simulink model "Backhoe_TiltCyl_Valve_Variants"  (R2016a)
settings: Solver=ode23t  StartTime=0.0  StopTime=60  MaxStep=0.01  RelTol=1e-3
PostLoadFcn:
  | warning off Simulink:Engine:UsingDefaultMaxStepSize
  | warning off Simulink:blocks:MatchingFromNotFound
  | warning off Simulink:Engine:SaveWithParameterizedLinks_Warning
  | warning off Simulink:Engine:SolverMinStepNonlinearIterWarnForDAE
model workspace (MAT data in the model file):
  cylinderGray = [0.6 0.6 0.6]
  darkOrange = [0.8 0.5 0]
  glassBlue = [0.2 0.2 1]
  gray = [0.3 0.3 0.3]
  orange = [0.8 0.65 0]
  pistonGray = [0.4 0.4 0.4]
  rhoGlass = 2500
  rhoRubber = 1500
  rhoSteel = 7800
  tireBlack = [0.1 0.1 0.1]
  wheelGray = [0.6 0.6 0.6]
  yellow = [0.8 0.8 0]
undefined symbols (not defined in the file or in its folder): BH_Param, sigbuilder_block, X, Y, Z
libraries: sm_lib x54, fl_lib x15, Backhoe_Lib x15, nesl_utility x7, sh_lib x4, Custom_Valve_Choices_Lib x1
(part 1 of 2)
Description:
  | Copyright 2014-2016 The MathWorks, Inc.
settings Model: Creator=smiller  LastModifiedBy=smiller
settings DataIOCC: LimitDataPoints=on  SaveFormat=Array
settings OptimizationCC: ExpressionDepthLimit=2147483647
settings DebuggingCC: UnderspecifiedInitializationDetection=Classic  MergeDetectMultiDrivingBlocksExec=none  SolverPrmCheckMsg=warning  AllowSymbolicDim=off  StateNameClashWarn=warning
settings HardwareCC: ProdBitPerPointer=32  ProdLargestAtomicFloat=None  ProdIntDivRoundTo=Undefined  ProdEndianess=Unspecified  ProdWordSize=32  ProdHWDeviceType=32-bit Generic
settings ModelReferenceCC: PropagateSignalLabelsOutOfModel=off
settings ConfigComp: CovModelRefEnable=Off  CovSFcnEnable=off
settings ConfigurationSet: Description=SimMechanics 2G
settings ExplorerConfigSet: InternalSimMechanicsExplorerSettings="<ExplorerConfiguration><canonicalview>default</canonicalview><TilePanel><TileInfo><Tiles Columns=\"1\" Count=\"1\" Rows=\"1\"><Column Left=\"2\" Weight=\"1\"/><Column Left=\"516\"/><Row Top=\"2\" Weight=\"1\"/><Row Top=\"405\"/><Tile Height=\"1\" Width=\"1\" X=\"0\" Y=\"0\"/></Tiles></TileInfo><SceneInfo><SceneViewer><BGColor><R>0.60000002384185791</R><G>0.60000002384185791</G><B>0.60000002384185791</B></BGColor><Camera><Position><X>0.52872575952314227</X><Y>-5.2039035895766403</Y><Z>-12.054682087754447</Z></Position><Center><X>2.5552113476516021</X><Y>-1.1721933566146352</Y><Z>-0.012277392551881244</Z></Center><Up><X>0.81449776203546786</X><Y>-0.5774326892391981</Y><Z>0.056257310966686652</Z></Up><Left>-3.995501128607974</Left><Right>3.995501128607974</Right><Bottom>-4.6400630968244965</Bottom><Top>4.6400630968244965</Top></Camera></SceneViewer></SceneInfo></TilePanel></ExplorerConfiguration>"

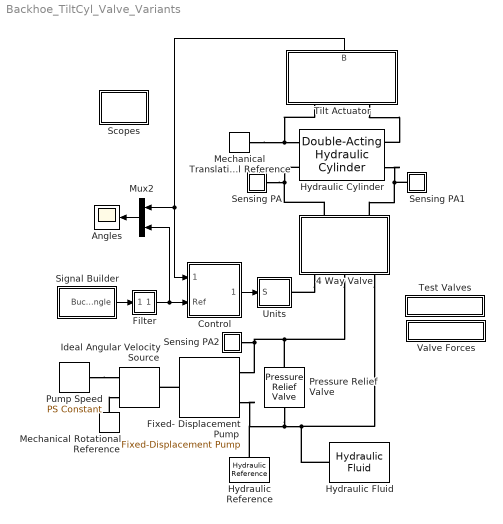
== system Backhoe_TiltCyl_Valve_Variants ==
  4 Way Valve : Subsystem  BlockChoice=Ideal
      link override Mech Spool/Orifices: BlockChoice=No Force
      link override Servovalve Center: pump_spool_orifice_area=1  ctr_spr_stiffness=360000  spool_damping=162*2
      link override Servovalve Center/Valve/Orifices: BlockChoice=No Force
      link override Servovalve Flapper/Valve/Orifices: BlockChoice=No Force
      settings: AttributesFormatString=%<BlockChoice>  TemplateBlock=Custom_Valve_Choices_Lib/4 Way Valve  MemberBlocks=Ideal,Mech Spool,Servovalve Center,Servovalve Flapper
      mask Display: disp(' ');
  Angles : Scope
  Control : Subsystem  mask(PID Controller){upperLim=10, lowerLim=-120, Kp=10, Ki=0.2, Kd=0.2, N=100}
      mask prompts: upperLim "Upper Limit [deg]"; lowerLim "Lower Limit [deg]"
      mask help: This block takes in a reference angle and measured angle, and uses a PID Controller with saturation to give a control command.
  Filter : Subsystem  mask{b=1e-1, x_initial=0}
      mask prompts: b "Filter time constant"; x_initial "Initial Output"
  Fixed- Displacement Pump : sh_lib/Pumps and Motors/Fixed-Displacement Pump  D=BH_Param.Hydraulic.Pump.Displacement m^3/rad  efficiency_vol=BH_Param.Hydraulic.Pump.Vol_Eff  efficiency_tot=BH_Param.Hydraulic.Pump.Total_Eff  pr_nominal=BH_Param.Hydraulic.Pump.Nominal_Pressure Pa  w_nominal=BH_Param.Hydraulic.Pump.Nominal_Ang_Vel rad/s  visc_nominal=BH_Param.Hydraulic.Pump.Nominal_Kin_Visc cSt  dens_nominal=900 kg/m^3
  Hydraulic Reference : fl_lib/Hydraulic/Hydraulic Elements/Hydraulic Reference
  Hydraulic Cylinder : sh_lib/Hydraulic Cylinders/Double-Acting Hydraulic Cylinder  Tag=Factory Generic  area_A=BH_Param.Tilt_Actuator.Cylinder.Area_A m^2  area_B=BH_Param.Tilt_Actuator.Cylinder.Area_B m^2  stroke=BH_Param.Tilt_Actuator.Cylinder.Stroke m  init_pos=BH_Param.Tilt_Actuator.Cylinder.x0 m  dead_vol_A=BH_Param.Tilt_Actuator.Cylinder.DeadVol_A m^3  dead_vol_B=BH_Param.Tilt_Actuator.Cylinder.DeadVol_B m^3  init_pressure_A=BH_Param.Tilt_Actuator.Cylinder.PA0 Pa  init_pressure_B=1.17e7 Pa  k_sh=1.4  stiff=1e+06 N/m  D=150 N/(m/s)  or=2
  Hydraulic Fluid : sh_lib/Hydraulic Utilities/Hydraulic Fluid  DataSource=1  SelFluid=9  SysTemp=50  TrapAir=0.004  ViscDerFactor=1  range_error=2
  Ideal Angular Velocity Source : fl_lib/Mechanical/Mechanical Sources/Ideal Angular Velocity Source
  Mechanical Rotational Reference : fl_lib/Mechanical/Rotational Elements/Mechanical Rotational Reference
  Mechanical Translational Reference : fl_lib/Mechanical/Translational Elements/Mechanical Translational Reference  Tag=Factory Generic
  Mux2 : Mux  Inputs=2
  Pressure Relief Valve : sh_lib/Valves/Pressure Control Valves/Pressure Relief Valve  area_max=BH_Param.Hydraulic.PRV.Max_Area m^2  pres_set=BH_Param.Hydraulic.PRV.Pressure_Set Pa  reg_range=BH_Param.Hydraulic.PRV.Pressure_Rng Pa  C_d=BH_Param.Hydraulic.PRV.Flow_Disch_Coeff  Re_cr=BH_Param.Hydraulic.PRV.Re_Critical  A_leak=BH_Param.Hydraulic.PRV.Leakage_Area m^2  dynamic=0  tau=0.1 s  area_init=1e-12 m^2
  Pump Speed : fl_lib/Physical Signals/Sources/PS Constant  constant=188
  Scopes : Subsystem
  Sensing PA : Subsystem
      mask Display: disp('S')
  Sensing PA1 : Subsystem
      mask Display: disp('S')
  Sensing PA2 : Subsystem
      mask Display: disp('S')
  Signal Builder : Subsystem  Tag=STV Subsys  LoadFcn=sigbuilder_block('load');  StartFcn=sigbuilder_block('start');  StopFcn=sigbuilder_block('stop');  ClipboardFcn=sigbuilder_block('clipboard');  mask(Sigbuilder block){}
      mask help: Simulink:masks:SigbuilderBlock_MD
      mask init:
      | if ~strcmp(get_param(bdroot(gcbh),'SimulationStatus'),'stopped') tuvar = sigbuilder_block('maskInit'); end
      settings: CopyFcn=sigbuilder_block('copy');  DeleteFcn=sigbuilder_block('delete');  ModelCloseFcn=sigbuilder_block('modelClose');  PreSaveFcn=sigbuilder_block('preSave');  PauseFcn=sigbuilder_block('pause');  ContinueFcn=sigbuilder_block('continue');  NameChangeFcn=sigbuilder_block('namechange');  OpenFcn=sigbuilder_block('open',[5.58621 9.31034 624.414 408.414 ]);  CloseFcn=sigbuilder_block('close');
      mask Display: plot(0, 0, 100, 100,[2, 2, 32, 32, 2], [68, 8, 8, 68, 68],[32, 2], [38, 38], [32, 19, 2],[53, 60, 44], [32, 17, 17, 2],[16, 16, 31, 31]);txt = getActiveGroup(gcbh);text(2, 100, txt,'verticalAlignment', 'top');
  Test Valves : Subsystem
      settings: OpenFcn=Custom_Valve_Test_Valves
      mask Display: disp('Test Valves')
  Tilt Actuator : Subsystem
      mask Display:
      | image(imread('Backhoe_Tilt_Actuator_IMAGE.jpg'));
      | port_label('lconn',1,'C');
      | port_label('lconn',2,'R');
      | port_label('output',1,'B');
  Units : Subsystem
  Valve Forces : Subsystem
      settings: OpenFcn=Custom_Valve_Test_Forces
      mask Display: disp('Valve Forces')
  wires:
  Tilt Actuator/1(B) -> Mux2/1, Control/1(Meas)
  Control/1(Cmd) -> Units/1(S)
  Mux2/1 -> Angles/1
  Signal Builder/1(Bucket Angle) -> Filter/1(In1)
  Filter/1(Out1) -> Mux2/2, Control/2(Ref)
  connections:
  4 Way Valve/RConn2 -- Pressure Relief Valve/LConn1 -- Fixed- Displacement Pump/RConn1 -- Sensing PA2/LConn1
  Pressure Relief Valve/RConn1 -- Fixed- Displacement Pump/RConn2 -- Hydraulic Reference/LConn1 -- Hydraulic Fluid/RConn1 -- 4 Way Valve/RConn3
  Mechanical Rotational Reference/LConn1 -- Ideal Angular Velocity Source/RConn2
  Fixed- Displacement Pump/LConn1 -- Ideal Angular Velocity Source/LConn1
  Pump Speed/RConn1 -- Ideal Angular Velocity Source/RConn1
  Sensing PA1/LConn1 -- 4 Way Valve/LConn2 -- Hydraulic Cylinder/RConn2
  Hydraulic Cylinder/LConn1 -- Tilt Actuator/LConn1 -- Mechanical Translational Reference/LConn1
  Hydraulic Cylinder/LConn2 -- 4 Way Valve/LConn1 -- Sensing PA/LConn1
  Tilt Actuator/LConn2 -- Hydraulic Cylinder/RConn1
  4 Way Valve/RConn1 -- Units/RConn1

== system Backhoe_TiltCyl_Valve_Variants/4 Way Valve ==
  Ideal : Custom_Valve_Choices_Lib/Ideal  orifice_width=24.5  max_spool_travel=0.005  x0_orifice_PA=0  x0_orifice_PB=0  x0_orifice_AT=0  x0_orifice_BT=0
  Port_A : PMIOPort  Port=1  Side=Left
  Port_B : PMIOPort  Port=2  Side=Left
  Port_S : PMIOPort  Port=3  Side=Right
  Port_P : PMIOPort  Port=4  Side=Right
  Port_T : PMIOPort  Port=5  Side=Right
  connections:
  Ideal/LConn1 -- Port_A/RConn1
  Ideal/LConn2 -- Port_B/RConn1
  Ideal/RConn1 -- Port_S/RConn1
  Ideal/RConn2 -- Port_P/RConn1
  Ideal/RConn3 -- Port_T/RConn1

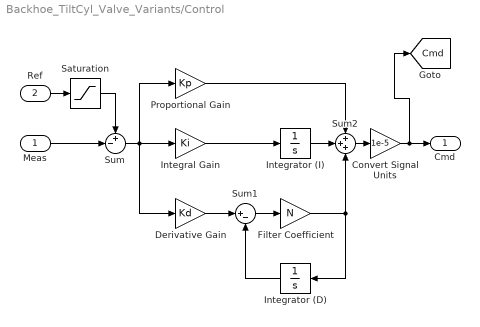
== system Backhoe_TiltCyl_Valve_Variants/Control ==
  Meas : Inport
  Ref : Inport  Port=2
  Convert Signal Units : Gain  Gain=1e-5
  Derivative Gain : Gain  Gain=Kd
  Filter Coefficient : Gain  Gain=N
  Integral Gain : Gain  Gain=Ki
  Integrator (D) : Integrator
  Integrator (I) : Integrator
  Proportional Gain : Gain  Gain=Kp
  Saturation : Saturate  UpperLimit=upperLim  LowerLimit=lowerLim
  Sum : Sum  Inputs=+-|
  Sum1 : Sum  Inputs=|+-
  Sum2 : Sum  Inputs=+++
  Cmd : Outport
  tag scope: Cmd=global
  wires:
  Saturation/1 -> Sum/1
  Meas/1 -> Sum/2
  Ref/1 -> Saturation/1
  Sum/1 -> Integral Gain/1, Proportional Gain/1, Derivative Gain/1
  Sum2/1 -> Convert Signal Units/1
  Integrator (I)/1 -> Sum2/2
  Integrator (D)/1 -> Sum1/2
  Filter Coefficient/1 -> Integrator (D)/1, Sum2/3
  Sum1/1 -> Filter Coefficient/1
  Derivative Gain/1 -> Sum1/1
  Integral Gain/1 -> Integrator (I)/1
  Proportional Gain/1 -> Sum2/1
  Convert Signal Units/1 -> [Cmd], Cmd/1

== system Backhoe_TiltCyl_Valve_Variants/Filter ==
  In1 : Inport
  Gain : Gain  Gain=1/b
  Integrator : Integrator  InitialCondition=x_initial
  Sum : Sum  Inputs=|+-
  Out1 : Outport
  wires:
  Gain/1 -> Integrator/1
  Integrator/1 -> Out1/1, Sum/2
  In1/1 -> Sum/1
  Sum/1 -> Gain/1

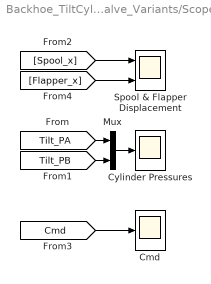
== system Backhoe_TiltCyl_Valve_Variants/Scopes ==
  Cmd : Scope
  Cylinder Pressures : Scope
  Mux : Mux  Inputs=2
  Spool & Flapper Displacement : Scope  NumInputPorts=2
  wires:
  [Spool_x] -> Spool & Flapper Displacement/1
  [Flapper_x] -> Spool & Flapper Displacement/2
  [Tilt_PB] -> Mux/2
  [Tilt_PA] -> Mux/1
  Mux/1 -> Cylinder Pressures/1
  [Cmd] -> Cmd/1

== system Backhoe_TiltCyl_Valve_Variants/Sensing PA ==
  Hydraulic Pressure Sensor : fl_lib/Hydraulic/Hydraulic Sensors/Hydraulic Pressure Sensor
  Hydraulic Reference1 : fl_lib/Hydraulic/Hydraulic Elements/Hydraulic Reference
  PS-Simulink Converter1 : nesl_utility/PS-Simulink Converter  PhysicalDomain=network_engine_domain  SubClassName=ps_output  LeftPortType=input  RightPortType=output  PseudoPeriodic=off  Frequencies=[]  Unit=1  AffineConversion=off
  A : PMIOPort  Port=1  Side=Left
  tag scope: Tilt_PA=global
  wires:
  PS-Simulink Converter1/1 -> [Tilt_PA]
  connections:
  PS-Simulink Converter1/LConn1 -- Hydraulic Pressure Sensor/RConn2
  Hydraulic Reference1/LConn1 -- Hydraulic Pressure Sensor/RConn1
  Hydraulic Pressure Sensor/LConn1 -- A/RConn1

== system Backhoe_TiltCyl_Valve_Variants/Sensing PA1 ==
  Hydraulic Pressure Sensor : fl_lib/Hydraulic/Hydraulic Sensors/Hydraulic Pressure Sensor
  Hydraulic Reference1 : fl_lib/Hydraulic/Hydraulic Elements/Hydraulic Reference
  PS-Simulink Converter1 : nesl_utility/PS-Simulink Converter  PhysicalDomain=network_engine_domain  SubClassName=ps_output  LeftPortType=input  RightPortType=output  PseudoPeriodic=off  Frequencies=[]  Unit=1  AffineConversion=off
  A : PMIOPort  Port=1  Side=Left
  tag scope: Tilt_PB=global
  wires:
  PS-Simulink Converter1/1 -> [Tilt_PB]
  connections:
  Hydraulic Pressure Sensor/LConn1 -- A/RConn1
  Hydraulic Reference1/LConn1 -- Hydraulic Pressure Sensor/RConn1
  PS-Simulink Converter1/LConn1 -- Hydraulic Pressure Sensor/RConn2

== system Backhoe_TiltCyl_Valve_Variants/Sensing PA2 ==
  Hydraulic Pressure Sensor : fl_lib/Hydraulic/Hydraulic Sensors/Hydraulic Pressure Sensor
  Hydraulic Reference1 : fl_lib/Hydraulic/Hydraulic Elements/Hydraulic Reference
  PS-Simulink Converter1 : nesl_utility/PS-Simulink Converter  PhysicalDomain=network_engine_domain  SubClassName=ps_output  LeftPortType=input  RightPortType=output  PseudoPeriodic=off  Frequencies=[]  Unit=1  AffineConversion=off
  A : PMIOPort  Port=1  Side=Left
  tag scope: Lift_PP=global
  wires:
  PS-Simulink Converter1/1 -> [Lift_PP]
  connections:
  PS-Simulink Converter1/LConn1 -- Hydraulic Pressure Sensor/RConn2
  Hydraulic Reference1/LConn1 -- Hydraulic Pressure Sensor/RConn1
  Hydraulic Pressure Sensor/LConn1 -- A/RConn1

== system Backhoe_TiltCyl_Valve_Variants/Signal Builder ==
  Demux : Demux  Tag=STV Demux  Outputs=1
  FromWs : FromWorkspace  Tag=STV FromWs  VariableName=tuvar  SampleTime=0  OutputAfterFinalValue=Holding final value
      SigBuilderData=|
      | common.afterFinalStr = 'Hold final value'
      | common.sampleTime = '0'
      | dataSet.timeRange = [0 60]
      | dataSet.name = 'Ref'
      | sbobj.Groups.Name = 'Ref'
      | sbobj.Groups.Signals.Name = 'Bucket Angle'
      | sbobj.Groups.Signals.XData = [0 7 11 24 28.5 40 42 51.5 53.5 60]
      | sbobj.Groups.Signals.YData = [0 0 -90 -90 0 0 -110 -110 0 0]
      | sbobj.Groups.TimeRange = [0 60]
  Bucket Angle : Outport  Tag=STV Outport
  wires:
  Demux/1 -> Bucket Angle/1
  FromWs/1 -> Demux/1

== system Backhoe_TiltCyl_Valve_Variants/Test Valves ==

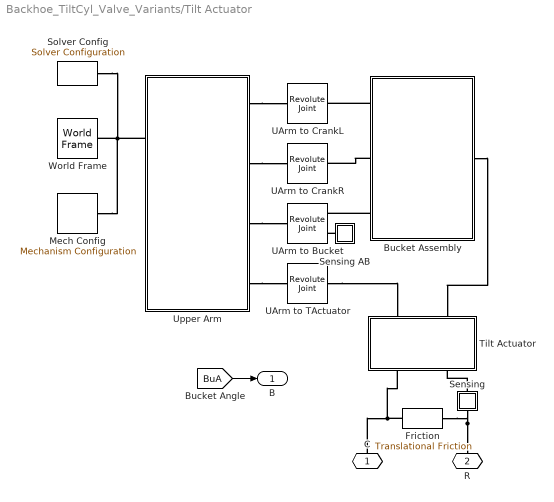
== system Backhoe_TiltCyl_Valve_Variants/Tilt Actuator ==
  Bucket Assembly : Subsystem
      mask Display:
      | image(imread('Backhoe_Arm_Bucket_Asy_IMAGE.JPG'));
      | port_label('lconn',1,'UAL');
      | port_label('lconn',2,'UAR');
      | port_label('lconn',3,'UA');
      | port_label('rconn',1,'TAct');
  Friction : fl_lib/Mechanical/Translational Elements/Translational Friction  brkwy_frc=BH_Param.Tilt_Actuator.Friction.Breakaway N  Col_frc=BH_Param.Tilt_Actuator.Friction.Coulomb N  visc_coef=BH_Param.Tilt_Actuator.Friction.Viscous N/(m/s)  trans_coef=10 s/m  vel_thr=1e-4 m/s  v_specify=off  v_priority=High  v=0 m/s  f_specify=off  f_priority=High  f=0 N
  Mech Config : sm_lib/Utilities/Mechanism Configuration  UniformGravity=Constant  GravityVector=[0 -9.81 0]  GravityUnits=m/s^2  LinearizationDelta=0.001
  Sensing : Subsystem
      mask Display: disp('S')
  Sensing AB : Subsystem
      mask Display: disp('S')
  Solver Config : nesl_utility/Solver Configuration  PhysicalDomain=network_engine_domain  SubClassName=solver  LeftPortType=input  RightPortType=generic  Accelerate=off  Tones=[]  Harmonics=[]  SimulateNoise=off  Profile=off  UseLocalSampling=off  EnableSwitchedLinearOptims=on  FrequencyDomain=off  UseCCode=off  RelTol=0.001  AbsTol=1e-06  MinStep=1e-09  ToWorkspace=off  RevertToSquareIcSolve=off  NumHomotopyIterations=100  PhasorMode=off  PhasorModeNumHarmonics=1  OverrideAbsTol=off  DoDC=off  ResidualTolerance=1e-9  UseLocalSolver=off  LocalSolverChoice=NE_BACKWARD_EULER_ADVANCER  LocalSolverSampleTime=.001  DoFixedCost=off  MaxNonlinIter=3  MaxModeIter=2  LinearAlgebra=Sparse  DelaysMemoryBudget=1024  AutomaticFiltering=on  FilteringTimeConstant=0.001
  Tilt Actuator : Subsystem  mask(Hydraulic Actuator){Lcyl=1.9, Rcyl=0.2, Lpist=1.9, Rpist=0.12, Lbase=0.65, Wbase=0.425, Rbp=0.075, Lbp=0.8, Whead=0.35, Lhead=0.65, Rhp=0.075, Lhp=0.9, circlePoints=25, cylColor=BH_Param.Colors.cylinderGray, rhoCyl=BH_Param.Densities.rhoSteel, pistColor=BH_Param.Colors.pistonGray, rhoPist=BH_Param.Densities.rhoSteel, connColor=BH_Param.Colors.gray, rhoConn=BH_Param.Densities.rhoSteel}
      mask prompts: Lcyl "Lcyl [m]"; Rcyl "Rcyl [m]"; Lpist "Lpist [m]"; Rpist "Rpist [m]"; Lbase "Lbase [m]"; Wbase "Wbase [m]"; Rbp "Rbp [m]"; Lbp "Lbp [m]"; Whead "Whead [m]"; Lhead "Lhead [m]"; Rhp "Rhp [m]"; Lhp "Lhp [m]"; circlePoints "Circle Mesh Resolution"; cylColor "Cylinder Color"; rhoCyl "Cylinder Density [kg/m^3]"; pistColor "Piston Color"; rhoPist "Piston Density [kg/m^3]"; connColor "Connector Color"; rhoConn "Connector Density [kg/m^3]"
      mask help:
      | Consists of the backhoe hydraulic actuator assembly.
      |
      | Zero piston displacement corresponds to the piston and cylinder centers of mass in the same position. Positive piston displacement is outward motion, and negative piston displacement is inward motion.
      |
      | Attachment points are:
      | C: Center of the Cylinder base bracket hole.
      | H: Center of the Piston Head bracket hole.
      | Both attachment points are configured for Revolute joints.
      |
      | The Simulink Signal input port supplies a Pressure value P (in Pa) to a Simscape hydraulic network.
      |
      | Click on Help to view a schematic of the hydraulic actuator, its configurable dimension parameters and attachment points (in red).
      mask init:
      | % Hollow Cylinder cross-section
      | cylSection = [];
      | 
      | for i = 0:2*circlePoints
      |     angle = (i/circlePoints)*pi;
      |     cylSection = [cylSection; Rcyl*cos(angle) Rcyl*sin(angle)];
      | end
      | 
      | for i = 0:2*circlePoints
      |     angle = -(i/circlePoints)*pi;
      |     cylSection = [cylSection; Rpist*cos(angle) Rpist*sin(angle)];
      | end
      mask Help: web('Backhoe_Actuator.html');
      mask Display:
      | image(imread('Backhoe_Arm_Actuator_IMAGE.jpg'));
      | port_label('lconn',1,'R');
      | port_label('lconn',2,'C');
      | port_label('rconn',1,'Cr');
      | port_label('rconn',2,'UA');
      | %port_label('input',1,'Cmd');
  UArm to Bucket : sm_lib/Joints/Revolute Joint  SenseConstraintForce=off  SenseConstraintForceX=off  SenseConstraintForceY=off  SenseConstraintForceZ=off  SenseConstraintTorque=off  SenseConstraintTorqueX=off  SenseConstraintTorqueY=off  SenseConstraintTorqueZ=off  SenseTotalForce=off  SenseTotalForceX=off  SenseTotalForceY=off  SenseTotalForceZ=off  SenseTotalTorque=off  SenseTotalTorqueX=off  SenseTotalTorqueY=off  SenseTotalTorqueZ=off  CompositeWrenchDir=FollowerOnBase  CompositeWrenchFrame=BaseFrame  EquilibriumPosition=0  EquilibriumPositionUnits=deg  SpringStiffness=0  SpringStiffnessUnits=N*m/deg  DampingCoefficient=0  DampingCoefficientUnits=N*m/(deg/s)  TorqueActuationMode=NoTorque  MotionActuationMode=ComputedMotion  SensePosition=on  SenseVelocity=off  SenseAcceleration=off  SenseTorqueForce=off  PositionTargetSpecify=on  PositionTargetPriority=High  PositionTargetValue=0  PositionTargetValueUnits=deg  VelocityTargetSpecify=off  VelocityTargetPriority=High  VelocityTargetValue=0  VelocityTargetValueUnits=deg/s
  UArm to CrankL : sm_lib/Joints/Revolute Joint  SenseConstraintForce=off  SenseConstraintForceX=off  SenseConstraintForceY=off  SenseConstraintForceZ=off  SenseConstraintTorque=off  SenseConstraintTorqueX=off  SenseConstraintTorqueY=off  SenseConstraintTorqueZ=off  SenseTotalForce=off  SenseTotalForceX=off  SenseTotalForceY=off  SenseTotalForceZ=off  SenseTotalTorque=off  SenseTotalTorqueX=off  SenseTotalTorqueY=off  SenseTotalTorqueZ=off  CompositeWrenchDir=FollowerOnBase  CompositeWrenchFrame=BaseFrame  EquilibriumPosition=0  EquilibriumPositionUnits=deg  SpringStiffness=0  SpringStiffnessUnits=N*m/deg  DampingCoefficient=0  DampingCoefficientUnits=N*m/(deg/s)  TorqueActuationMode=NoTorque  MotionActuationMode=ComputedMotion  SensePosition=off  SenseVelocity=off  SenseAcceleration=off  SenseTorqueForce=off  PositionTargetSpecify=off  PositionTargetPriority=Low  PositionTargetValue=-150  PositionTargetValueUnits=deg  VelocityTargetSpecify=off  VelocityTargetPriority=High  VelocityTargetValue=0  VelocityTargetValueUnits=deg/s
  UArm to CrankR : sm_lib/Joints/Revolute Joint  SenseConstraintForce=off  SenseConstraintForceX=off  SenseConstraintForceY=off  SenseConstraintForceZ=off  SenseConstraintTorque=off  SenseConstraintTorqueX=off  SenseConstraintTorqueY=off  SenseConstraintTorqueZ=off  SenseTotalForce=off  SenseTotalForceX=off  SenseTotalForceY=off  SenseTotalForceZ=off  SenseTotalTorque=off  SenseTotalTorqueX=off  SenseTotalTorqueY=off  SenseTotalTorqueZ=off  CompositeWrenchDir=FollowerOnBase  CompositeWrenchFrame=BaseFrame  EquilibriumPosition=0  EquilibriumPositionUnits=deg  SpringStiffness=0  SpringStiffnessUnits=N*m/deg  DampingCoefficient=0  DampingCoefficientUnits=N*m/(deg/s)  TorqueActuationMode=NoTorque  MotionActuationMode=ComputedMotion  SensePosition=off  SenseVelocity=off  SenseAcceleration=off  SenseTorqueForce=off  PositionTargetSpecify=off  PositionTargetPriority=High  PositionTargetValue=0  PositionTargetValueUnits=deg  VelocityTargetSpecify=off  VelocityTargetPriority=High  VelocityTargetValue=0  VelocityTargetValueUnits=deg/s
  UArm to TActuator : sm_lib/Joints/Revolute Joint  SenseConstraintForce=off  SenseConstraintForceX=off  SenseConstraintForceY=off  SenseConstraintForceZ=off  SenseConstraintTorque=off  SenseConstraintTorqueX=off  SenseConstraintTorqueY=off  SenseConstraintTorqueZ=off  SenseTotalForce=off  SenseTotalForceX=off  SenseTotalForceY=off  SenseTotalForceZ=off  SenseTotalTorque=off  SenseTotalTorqueX=off  SenseTotalTorqueY=off  SenseTotalTorqueZ=off  CompositeWrenchDir=FollowerOnBase  CompositeWrenchFrame=BaseFrame  EquilibriumPosition=0  EquilibriumPositionUnits=deg  SpringStiffness=0  SpringStiffnessUnits=N*m/deg  DampingCoefficient=0  DampingCoefficientUnits=N*m/(deg/s)  TorqueActuationMode=NoTorque  MotionActuationMode=ComputedMotion  SensePosition=off  SenseVelocity=off  SenseAcceleration=off  SenseTorqueForce=off  PositionTargetSpecify=on  PositionTargetPriority=Low  PositionTargetValue=-90  PositionTargetValueUnits=deg  VelocityTargetSpecify=off  VelocityTargetPriority=High  VelocityTargetValue=0  VelocityTargetValueUnits=deg/s
  Upper Arm : Subsystem
      mask Display:
      | image(imread('Backhoe_Arm_Upper_IMAGE.JPG'));
      | port_label('lconn',1,'LA');
      | port_label('lconn',2,'RAct');
      | port_label('rconn',1,'CrL');
      | port_label('rconn',2,'CrR');
      | port_label('rconn',3,'B');
      | port_label('rconn',4,'TAct');
  World Frame : sm_lib/Frames and Transforms/World Frame
  C : PMIOPort  Port=1  Side=Left
  R : PMIOPort  Port=2  Side=Left
  B : Outport
  wires:
  [BuA] -> B/1
  connections:
  C/RConn1 -- Tilt Actuator/LConn2 -- Friction/RConn1
  Bucket Assembly/LConn1 -- UArm to CrankL/RConn1
  Sensing AB/LConn1 -- UArm to Bucket/RConn2
  Upper Arm/RConn1 -- UArm to CrankL/LConn1
  Upper Arm/RConn4 -- UArm to TActuator/LConn1
  Upper Arm/RConn2 -- UArm to CrankR/LConn1
  Bucket Assembly/LConn2 -- UArm to CrankR/RConn1
  Bucket Assembly/RConn1 -- Tilt Actuator/RConn1
  Friction/LConn1 -- Sensing/LConn1 -- R/RConn1
  UArm to TActuator/RConn1 -- Tilt Actuator/RConn2
  Bucket Assembly/LConn3 -- UArm to Bucket/RConn1
  Upper Arm/RConn3 -- UArm to Bucket/LConn1
  Mech Config/RConn1 -- Upper Arm/LConn1 -- Solver Config/RConn1 -- World Frame/RConn1
  Sensing/RConn1 -- Tilt Actuator/LConn1

== system Backhoe_TiltCyl_Valve_Variants/Units ==
  S : Inport
  Simulink-PS Converter : nesl_utility/Simulink-PS Converter  PhysicalDomain=network_engine_domain  SubClassName=ps_input  LeftPortType=input  RightPortType=output  PseudoPeriodic=off  Frequencies=[]  NoiseDistribution=none  NoiseParameters=[]  Unit=1  AffineConversion=off  InputFiltering=off  SimscapeFilterOrder=1  InputFilterTimeConstant=.001  UdotUserProvided=0
  PS : PMIOPort  Port=1  Side=Right
  wires:
  S/1 -> Simulink-PS Converter/1
  connections:
  Simulink-PS Converter/RConn1 -- PS/RConn1

== system Backhoe_TiltCyl_Valve_Variants/Valve Forces ==

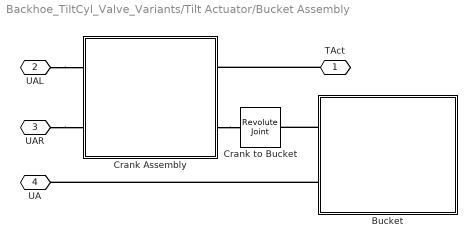
== system Backhoe_TiltCyl_Valve_Variants/Tilt Actuator/Bucket Assembly ==
  Bucket : Subsystem  mask(Bucket){plateSide=1.2, plateFilletR=0.2, plateDist=1.2, plateWidth=0.2, plateHoleR=0.075, bucketHeight=2, bucketLength=2, bucketThickness=0.05, bucketUpper=1.3, bucketLower=2, chordAngle=pi/6, toothLength=0.25, toothWidth=0.2, toothTip=0.025, circlePoints=45, bucketColor=yellow, bracketColor=yellow, rho=rhoSteel}
      mask prompts: plateSide "Wplate [m]"; plateFilletR "Rfillet [m]"; plateDist "Dplate [m]"; plateWidth "Tplate [m]"; plateHoleR "Rpin [m]"; bucketHeight "Hbucket [m]"; bucketLength "Wbucket [m]"; bucketThickness "Tbucket [m]"; bucketUpper "Wupper [m]"; bucketLower "Wlower [m]"; chordAngle "alpha [radians]"; toothLength "Ltooth [m]"; toothWidth "Wtooth [m]"; toothTip "Ttooth [m]"; circlePoints "Circle Mesh Resolution"; bucketColor "Bucket Color"; bracketColor "Bracket Color"; rho "Density [kg/m^3]"
      mask help:
      | Consists of the backhoe bucket assembly with attachment frame.
      |
      | Attachment points are:
      | CA: Center point of the Crank Arm link pin.
      | UA: Center Point of the Upper Arm link pin.
      | Both points are configured for Revolute joints.
      |
      | Click on Help to view a schematic of the bucket, its configurable dimension parameters and attachment points (in red).
      mask init:
      | bucketRadius = bucketHeight/(2*cos(chordAngle));
      | 
      | % Bucket Back
      | bucketBack = [];
      | % Outer wall
      | for i = 0:circlePoints;
      |    angle = (-pi/2+chordAngle) + (pi - 2*chordAngle)*(i/circlePoints);
      |    bucketBack = [bucketBack; ...
      |        (bucketRadius*cos(angle)-bucketRadius*sin(chordAngle)) ...
      |         bucketRadius*sin(angle)];
      | end
      | 
      | % Inner Wall
      | beta = acos( ( (bucketRadius*cos(chordAngle) - bucketThickness/cos(chordAngle)) ...
      |                    /(bucketRadius-bucketThickness)) );
      | for i = 0:circlePoints;
      |    angle = (pi/2 - beta) - (pi-2*beta)*(i/circlePoints);
      |    bucketBack = [bucketBack; ...
      |        ((bucketRadius-bucketThickness)*cos(angle)-bucketRadius*sin(chordAngle)) ... 
      |        (bucketRadius-bucketThickness)*sin(angle)];
      | end
      | 
      | bucketBack = [bucketBack; ...
      |               -bucketLower -(bucketHeight/2-bucketThickness);...
      |               -bucketLower -bucketHeight/2];
      |           
      | % Uncomment below to plot the cross-sections. 
      | % close all
      | % figure
      | % plot(bucketBack(:,1),bucketBack(:,2));
      mask Help: web('Backhoe_Bucket.html');
      mask Display:
      | image(imread('Backhoe_Bucket_IMAGE.png'));
      | port_label('rconn',1,'CA');
      | port_label('rconn',2,'UA');
  Crank Assembly : Subsystem  mask(Crank Assembly){LC1=1.5, WC1=0.4, TC1=0.2, DH1=1.1, RH1=0.075, LC2=1.75, WC2=0.4, TC2=0.15, DH2=1.35, RH2=0.075, DC2=0.7, Wbar=0.8, Lpin=1.3, Rpin=0.075, circlePoints=25, color1=orange, color2=darkOrange, rho1=rhoSteel, rho2=rhoSteel}
      mask prompts: LC1 "LC1 [m]"; WC1 "WC1 [m]"; TC1 "TC1 [m]"; DH1 "DH1 [m]"; RH1 "RH1 [m]"; LC2 "LC2 [m]"; WC2 "WC2 [m]"; TC2 "TC2 [m]"; DH2 "DH2 [m]"; RH2 "RH2 [m]"; DC2 "DC2 [m]"; Wbar "Upper Arm Width, Wbar [m]"; Lpin "Lpin [m]"; Rpin "Rpin [m]"; circlePoints "Circle Mesh Resolution"; color1 "Color"; color2 "Color"; rho1 "Density [kg/m^3]"; rho2 "Density [kg/m^3]"
      mask help:
      | Consists of the backhoe crank assembly that connects the upper arm and the bucket. Crank 1 attaches to either side of the upper arm linkage, and Crank 2 connects Crank 1 and the Bucket.
      |
      | Attachment points are:
      | AL: Arm attachment (Left).
      | AR: Arm attachment (Right).
      | B: Bucket attachment.
      | P: Piston attachment.
      | All attachment points are configured for Revolute joints.
      |
      | Click on Help to view a schematic of the crank assembly, its configurable dimension parameters and attachment points (in red).
      mask Help: web('Backhoe_Crank.html');
      mask Display:
      | image(imread('Backhoe_Crankassembly_IMAGE.png'));
      | port_label('rconn',1,'B');
      | port_label('rconn',2,'P');
      | port_label('lconn',1,'AL');
      | port_label('lconn',2,'AR');
  Crank to Bucket : sm_lib/Joints/Revolute Joint  SenseConstraintForce=off  SenseConstraintForceX=off  SenseConstraintForceY=off  SenseConstraintForceZ=off  SenseConstraintTorque=off  SenseConstraintTorqueX=off  SenseConstraintTorqueY=off  SenseConstraintTorqueZ=off  SenseTotalForce=off  SenseTotalForceX=off  SenseTotalForceY=off  SenseTotalForceZ=off  SenseTotalTorque=off  SenseTotalTorqueX=off  SenseTotalTorqueY=off  SenseTotalTorqueZ=off  CompositeWrenchDir=FollowerOnBase  CompositeWrenchFrame=BaseFrame  EquilibriumPosition=0  EquilibriumPositionUnits=deg  SpringStiffness=0  SpringStiffnessUnits=N*m/deg  DampingCoefficient=0  DampingCoefficientUnits=N*m/(deg/s)  TorqueActuationMode=NoTorque  MotionActuationMode=ComputedMotion  SensePosition=off  SenseVelocity=off  SenseAcceleration=off  SenseTorqueForce=off  PositionTargetSpecify=off  PositionTargetPriority=Low  PositionTargetValue=0  PositionTargetValueUnits=deg  VelocityTargetSpecify=off  VelocityTargetPriority=High  VelocityTargetValue=0  VelocityTargetValueUnits=deg/s
  TAct : PMIOPort  Port=1  Side=Right
  UAL : PMIOPort  Port=2  Side=Left
  UAR : PMIOPort  Port=3  Side=Left
  UA : PMIOPort  Port=4  Side=Left
  connections:
  Bucket/RConn1 -- Crank to Bucket/RConn1
  Crank Assembly/RConn2 -- Crank to Bucket/LConn1
  Bucket/RConn2 -- UA/RConn1
  UAL/RConn1 -- Crank Assembly/LConn1
  UAR/RConn1 -- Crank Assembly/LConn2
  TAct/RConn1 -- Crank Assembly/RConn1

== system Backhoe_TiltCyl_Valve_Variants/Tilt Actuator/Sensing ==
  Ideal Force Sensor : fl_lib/Mechanical/Mechanical Sensors/Ideal Force Sensor
  PS-Simulink Converter : nesl_utility/PS-Simulink Converter  PhysicalDomain=network_engine_domain  SubClassName=ps_output  LeftPortType=input  RightPortType=output  PseudoPeriodic=off  Frequencies=[]  Unit=1  AffineConversion=off
  C : PMIOPort  Port=1  Side=Right
  R : PMIOPort  Port=2  Side=Left
  tag scope: Tilt_Act_F=global
  wires:
  PS-Simulink Converter/1 -> [Tilt_Act_F]
  connections:
  PS-Simulink Converter/LConn1 -- Ideal Force Sensor/RConn2
  Ideal Force Sensor/RConn1 -- C/RConn1
  Ideal Force Sensor/LConn1 -- R/RConn1

== system Backhoe_TiltCyl_Valve_Variants/Tilt Actuator/Sensing AB ==
  PS-Simulink Converter Upper1 : nesl_utility/PS-Simulink Converter  PhysicalDomain=network_engine_domain  SubClassName=ps_output  LeftPortType=input  RightPortType=output  PseudoPeriodic=off  Frequencies=[]  Unit=deg  AffineConversion=off
  Conn1 : PMIOPort  Port=1  Side=Left
  tag scope: BuA=global
  wires:
  PS-Simulink Converter Upper1/1 -> [BuA]
  connections:
  PS-Simulink Converter Upper1/LConn1 -- Conn1/RConn1

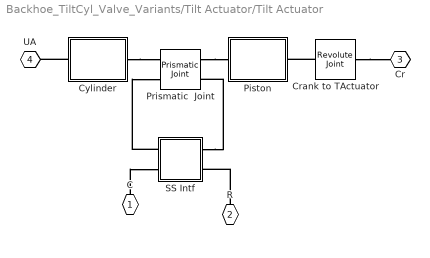
== system Backhoe_TiltCyl_Valve_Variants/Tilt Actuator/Tilt Actuator ==
  Crank to TActuator : sm_lib/Joints/Revolute Joint  SenseConstraintForce=off  SenseConstraintForceX=off  SenseConstraintForceY=off  SenseConstraintForceZ=off  SenseConstraintTorque=off  SenseConstraintTorqueX=off  SenseConstraintTorqueY=off  SenseConstraintTorqueZ=off  SenseTotalForce=off  SenseTotalForceX=off  SenseTotalForceY=off  SenseTotalForceZ=off  SenseTotalTorque=off  SenseTotalTorqueX=off  SenseTotalTorqueY=off  SenseTotalTorqueZ=off  CompositeWrenchDir=FollowerOnBase  CompositeWrenchFrame=BaseFrame  EquilibriumPosition=0  EquilibriumPositionUnits=deg  SpringStiffness=0  SpringStiffnessUnits=N*m/deg  DampingCoefficient=0  DampingCoefficientUnits=N*m/(deg/s)  TorqueActuationMode=NoTorque  MotionActuationMode=ComputedMotion  SensePosition=off  SenseVelocity=off  SenseAcceleration=off  SenseTorqueForce=off  PositionTargetSpecify=off  PositionTargetPriority=High  PositionTargetValue=0  PositionTargetValueUnits=deg  VelocityTargetSpecify=off  VelocityTargetPriority=High  VelocityTargetValue=0  VelocityTargetValueUnits=deg/s
  Cylinder : Subsystem
  Piston : Subsystem
  Prismatic  Joint : sm_lib/Joints/Prismatic Joint  SenseConstraintForce=off  SenseConstraintForceX=off  SenseConstraintForceY=off  SenseConstraintForceZ=off  SenseConstraintTorque=off  SenseConstraintTorqueX=off  SenseConstraintTorqueY=off  SenseConstraintTorqueZ=off  SenseTotalForce=off  SenseTotalForceX=off  SenseTotalForceY=off  SenseTotalForceZ=off  SenseTotalTorque=off  SenseTotalTorqueX=off  SenseTotalTorqueY=off  SenseTotalTorqueZ=off  CompositeWrenchDir=FollowerOnBase  CompositeWrenchFrame=BaseFrame  EquilibriumPosition=0  EquilibriumPositionUnits=m  SpringStiffness=0  SpringStiffnessUnits=N/m  DampingCoefficient=0  DampingCoefficientUnits=N/(m/s)  TorqueActuationMode=InputTorque  MotionActuationMode=ComputedMotion  SensePosition=off  SenseVelocity=on  SenseAcceleration=off  SenseTorqueForce=off  PositionTargetSpecify=off  PositionTargetPriority=Low  PositionTargetValue=0  PositionTargetValueUnits=m  VelocityTargetSpecify=off  VelocityTargetPriority=High  VelocityTargetValue=0  VelocityTargetValueUnits=m/s
  SS Intf : Subsystem
  C : PMIOPort  Port=1  Side=Left
  R : PMIOPort  Port=2  Side=Left
  Cr : PMIOPort  Port=3  Side=Right
  UA : PMIOPort  Port=4  Side=Right
  connections:
  Cylinder/RConn1 -- UA/RConn1
  Crank to TActuator/RConn1 -- Cr/RConn1
  Crank to TActuator/LConn1 -- Piston/RConn1
  Cylinder/LConn1 -- Prismatic  Joint/LConn1
  Prismatic  Joint/RConn1 -- Piston/LConn1
  SS Intf/LConn1 -- Prismatic  Joint/RConn2
  SS Intf/RConn1 -- Prismatic  Joint/LConn2
  C/RConn1 -- SS Intf/RConn2
  R/RConn1 -- SS Intf/LConn2

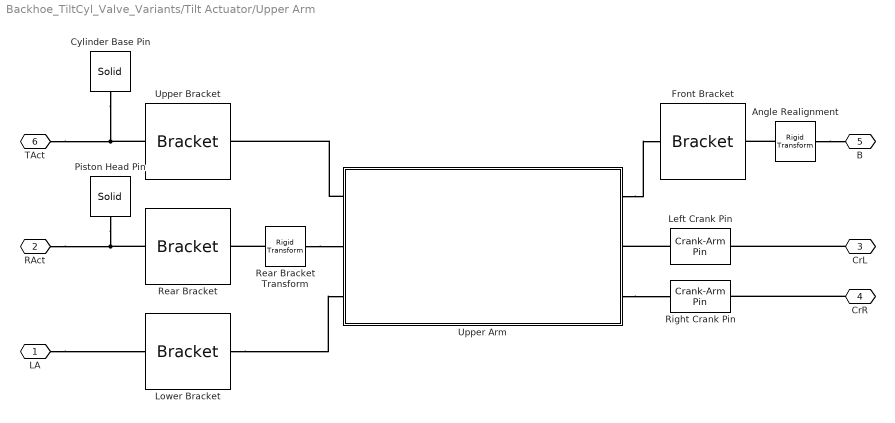
== system Backhoe_TiltCyl_Valve_Variants/Tilt Actuator/Upper Arm ==
  Angle Realignment : sm_lib/Frames and Transforms/Rigid Transform  TranslationMethod=None  TranslationLengthUnit=m  TranslationStandardAxis=+Z  TranslationStandardOffset=0  TranslationCartesianOffset=[0 0 0]  TranslationROffset=0  TranslationROffsetUnits=m  TranslationZOffset=0  TranslationZOffsetUnits=m  TranslationThetaOffset=0  TranslationThetaOffsetUnits=deg  RotationMethod=AlignedAxes  RotationAngleUnits=deg  RotationStandardAxis=-Z  RotationAngle=90  RotationArbitraryAxis=[0 0 1]  FollAlignAxisA=+X  BaseAlignAxisA=-Y  FollAlignAxisB=+Z  BaseAlignAxisB=+Z  RotationSequenceAxes=FollowerAxes  RotationSequence=XYX  RotationSequenceAngles=[0 0 0]  RotationSequenceAnglesUnits=deg  RotationMatrix=[1 0 0; 0 1 0; 0 0 1]
  Cylinder Base Pin : sm_lib/Body Elements/Solid  InertiaType=CalculateFromGeometry  Mass=1  MassUnits=kg  CenterOfMass=[0 0 0]  CenterOfMassUnits=m  MomentsOfInertia=[1 1 1]  MomentsOfInertiaUnits=kg*m^2  ProductsOfInertia=[0 0 0]  ProductsOfInertiaUnits=kg*m^2  DensityBased=on  Density=rhoSteel  DensityUnits=kg/(m^3)  DoExposeReferenceFrame=on  SerializedFrames=<Frames/>  GraphicType=FromGeometry  MarkerShape=Sphere  MarkerSize=10  MarkerSizeUnits=m  GraphicVisPropType=SimpleVisualProperties  GraphicDiffuseColor=gray  GraphicSpecularColor=[0.5 0.5 0.5 1.0]  GraphicAmbientColor=[0.15 0.15 0.15 1.0]  GraphicEmissiveColor=[0.0 0.0 0.0 1.0]  GraphicShininess=75  GraphicOpacity=1.0  GeometryShape=Cylinder  RectangleSize=[1 1]  RectangleSizeUnits=m  BrickDimensions=[3 0.5 0.5]  BrickDimensionUnits=m  CylinderRadius=0.075  CylinderRadiusUnits=m  CylinderLength=0.8  CylinderLengthUnits=m  SphereRadius=1  SphereRadiusUnits=m  EllipsoidRadii=[1 1 1]  EllipsoidRadiiUnits=m  ExtrusionCrossSection=[1 1; -1 1; -1 -1; 1 -1]  ExtrusionCrossSectionUnits=m  ExtrusionLength=1  ExtrusionLengthUnits=m  PolygonNumSides=3  PolygonOuterRadius=1  PolygonOuterRadiusUnits=m  ExtGeomFileType=STL  ExtGeomFileUnits=m  RevolutionCrossSection=[1 1; 1 -1; 2 -1; 2 1]  RevolutionCrossSectionUnits=m  RevolutionExtent=Full  RevolutionAngle=180  RevolutionAngleUnits=deg
  Front Bracket : Backhoe_Lib/Bracket  Hbracket=0.65  Wbracket=0.5  Tbracket=0.15  Dbracket=0.625  Hhole=0.4  Rhole=0.075  circlePoints=25  bracketColor=orange  rho=rhoSteel
  Left Crank Pin : Backhoe_Lib/Crank-Arm Pin  R=0.075  L=0.25  T=0.2  color=gray  rho=rhoSteel
  Lower Bracket : Backhoe_Lib/Bracket  Hbracket=0.75  Wbracket=0.75  Tbracket=0.15  Dbracket=0.75  Hhole=0.5  Rhole=0.075  circlePoints=25  bracketColor=orange  rho=rhoSteel
  Piston Head Pin : sm_lib/Body Elements/Solid  InertiaType=CalculateFromGeometry  Mass=1  MassUnits=kg  CenterOfMass=[0 0 0]  CenterOfMassUnits=m  MomentsOfInertia=[1 1 1]  MomentsOfInertiaUnits=kg*m^2  ProductsOfInertia=[0 0 0]  ProductsOfInertiaUnits=kg*m^2  DensityBased=on  Density=rhoSteel  DensityUnits=kg/(m^3)  DoExposeReferenceFrame=on  SerializedFrames=<Frames/>  GraphicType=FromGeometry  MarkerShape=Sphere  MarkerSize=10  MarkerSizeUnits=m  GraphicVisPropType=SimpleVisualProperties  GraphicDiffuseColor=gray  GraphicSpecularColor=[0.5 0.5 0.5 1.0]  GraphicAmbientColor=[0.15 0.15 0.15 1.0]  GraphicEmissiveColor=[0.0 0.0 0.0 1.0]  GraphicShininess=75  GraphicOpacity=1.0  GeometryShape=Cylinder  RectangleSize=[1 1]  RectangleSizeUnits=m  BrickDimensions=[1 1 1]  BrickDimensionUnits=m  CylinderRadius=0.075  CylinderRadiusUnits=m  CylinderLength=0.8  CylinderLengthUnits=m  SphereRadius=1  SphereRadiusUnits=m  EllipsoidRadii=[1 1 1]  EllipsoidRadiiUnits=m  ExtrusionCrossSection=[1 1; -1 1; -1 -1; 1 -1]  ExtrusionCrossSectionUnits=m  ExtrusionLength=1  ExtrusionLengthUnits=m  PolygonNumSides=3  PolygonOuterRadius=1  PolygonOuterRadiusUnits=m  ExtGeomFileType=STL  ExtGeomFileUnits=m  RevolutionCrossSection=[1 1; 1 -1; 2 -1; 2 1]  RevolutionCrossSectionUnits=m  RevolutionExtent=Full  RevolutionAngle=180  RevolutionAngleUnits=deg
  Rear Bracket : Backhoe_Lib/Bracket  Hbracket=0.75  Wbracket=0.75  Tbracket=0.15  Dbracket=0.75  Hhole=0.5  Rhole=0.075  circlePoints=25  bracketColor=orange  rho=rhoSteel
  Rear Bracket Transform : sm_lib/Frames and Transforms/Rigid Transform  TranslationMethod=None  TranslationLengthUnit=m  TranslationStandardAxis=+Z  TranslationStandardOffset=0.5  TranslationCartesianOffset=[ 0 0 0]  TranslationROffset=0  TranslationROffsetUnits=m  TranslationZOffset=0  TranslationZOffsetUnits=m  TranslationThetaOffset=0  TranslationThetaOffsetUnits=deg  RotationMethod=AlignedAxes  RotationAngleUnits=deg  RotationStandardAxis=+X  RotationAngle=90  RotationArbitraryAxis=[0 0 1]  FollAlignAxisA=+Z  BaseAlignAxisA=+Z  FollAlignAxisB=+Y  BaseAlignAxisB=-Y  RotationSequenceAxes=FollowerAxes  RotationSequence=XYX  RotationSequenceAngles=[0 0 0]  RotationSequenceAnglesUnits=deg  RotationMatrix=[1 0 0; 0 1 0; 0 0 1]
  Right Crank Pin : Backhoe_Lib/Crank-Arm Pin  R=0.075  L=0.25  T=0.2  color=gray  rho=rhoSteel
  Upper Arm : Subsystem  mask(Upper Arm){Lbar=6, Wbar=0.8, Tbar=0.85, L1=1.5, L2=1.5, L3=2.5, barFillet=0.1, numPoints=15, Tcrank=0.2, armColor=yellow, rho=rhoSteel}
      mask prompts: Lbar "Lbar [m]"; Wbar "Wbar [m]"; Tbar "Tbar [m]"; L1 "L1 [m]"; L2 "L2 [m]"; L3 "L3 [m]"; barFillet "Bar Fillet Radius [m]"; numPoints "Fillet Point Resolution"; Tcrank "Crank Arm Thickness [m]"; armColor "Arm Color"; rho "Density [kg/m^3]"
      mask help:
      | Consists of the backhoe upper arm and four attachment brackets -- front, rear, upper and lower.
      |
      | Attachment points are:
      | B: Bucket attachment.
      | CL: Crank arm attachment (Left).
      | CR: Crank arm attachment (Right).
      | BC: Bucket hydraulic actuator (Cylinder base).
      | LA: Lower Arm attachment.
      | UH: Upper arm hydraulic actuator (piston Head).
      | All attachment points are configured for Revolute joints.
      |
      | The lengths L1, L2 and L3 correspond to lengths measured from the center of the bar, as follows:
      | L1: Upper Bracket
      | L2: Lower Bracket
      | L3: Crank Attachment Points
      | The front and rear brackets are automatically placed at the center of the end faces of the upper arm bar.
      |
      | Click on Help to view a schematic of the upper arm, its configurable dimension parameters and attachment points (in red).
      mask init:
      | barSection = [Tbar/2 Wbar/2;  ...
      |              -Tbar/2 Wbar/2;  ...
      |              -Tbar/2 -Wbar/2; ...
      |               Tbar/2 -Wbar/2];
      | barSection = Extr_Data_Round_Corners(barSection,1:4,barFillet,numPoints);
      mask Help: web('Backhoe_Upperarm.html');
      mask Display:
      | image(imread('Backhoe_Upperbar_IMAGE.png'));
      | port_label('lconn',1,'CB');
      | port_label('lconn',2,'PH');
      | port_label('lconn',3,'LA');
      | port_label('rconn',1,'B');
      | port_label('rconn',2,'CL');
      | port_label('rconn',3,'CR');
  Upper Bracket : Backhoe_Lib/Bracket  Hbracket=0.75  Wbracket=0.75  Tbracket=0.15  Dbracket=0.75  Hhole=0.5  Rhole=0.075  circlePoints=25  bracketColor=orange  rho=rhoSteel
  LA : PMIOPort  Port=1  Side=Left
  RAct : PMIOPort  Port=2  Side=Left
  CrL : PMIOPort  Port=3  Side=Right
  CrR : PMIOPort  Port=4  Side=Right
  B : PMIOPort  Port=5  Side=Right
  TAct : PMIOPort  Port=6  Side=Right
  connections:
  Cylinder Base Pin/RConn1 -- Upper Bracket/RConn1 -- TAct/RConn1
  Piston Head Pin/RConn1 -- RAct/RConn1 -- Rear Bracket/RConn1
  Angle Realignment/LConn1 -- Front Bracket/RConn1
  LA/RConn1 -- Lower Bracket/RConn1
  CrL/RConn1 -- Left Crank Pin/LConn1
  CrR/RConn1 -- Right Crank Pin/LConn1
  Rear Bracket Transform/RConn1 -- Rear Bracket/LConn1
  Upper Arm/LConn1 -- Upper Bracket/LConn1
  Upper Arm/RConn1 -- Front Bracket/LConn1
  Upper Arm/RConn3 -- Right Crank Pin/RConn1
  Lower Bracket/LConn1 -- Upper Arm/LConn3
  Rear Bracket Transform/LConn1 -- Upper Arm/LConn2
  Left Crank Pin/RConn1 -- Upper Arm/RConn2
  Angle Realignment/RConn1 -- B/RConn1

== system Backhoe_TiltCyl_Valve_Variants/Tilt Actuator/Bucket Assembly/Bucket ==
  Arm Revolute Rotation : sm_lib/Frames and Transforms/Rigid Transform  TranslationMethod=None  TranslationLengthUnit=m  TranslationStandardAxis=+X  TranslationStandardOffset=0  TranslationCartesianOffset=[0 0 0]  TranslationROffset=0  TranslationROffsetUnits=m  TranslationZOffset=0  TranslationZOffsetUnits=m  TranslationThetaOffset=0  TranslationThetaOffsetUnits=deg  RotationMethod=AlignedAxes  RotationAngleUnits=deg  RotationStandardAxis=-Y  RotationAngle=180  RotationArbitraryAxis=[0 0 1]  FollAlignAxisA=+Y  BaseAlignAxisA=+Y  FollAlignAxisB=+X  BaseAlignAxisB=-X  RotationSequenceAxes=FollowerAxes  RotationSequence=XYX  RotationSequenceAngles=[0 0 0]  RotationSequenceAnglesUnits=deg  RotationMatrix=[1 0 0; 0 1 0; 0 0 1]
  Attachment Frame : Subsystem
      mask Display:
      | image(imread('Backhoe_Attach_IMAGE.png'));
      | port_label('lconn',1,'B');
      | port_label('rconn',1,'CA');
      | port_label('rconn',2,'UA');
  Bucket : Subsystem
      mask Display:
      | image(imread('Backhoe_Bucketcase_IMAGE.png'));
      | port_label('rconn',1,'AF');
  Crank Revolute Rotation : sm_lib/Frames and Transforms/Rigid Transform  TranslationMethod=None  TranslationLengthUnit=m  TranslationStandardAxis=+X  TranslationStandardOffset=0  TranslationCartesianOffset=[0 0 0]  TranslationROffset=0  TranslationROffsetUnits=m  TranslationZOffset=0  TranslationZOffsetUnits=m  TranslationThetaOffset=0  TranslationThetaOffsetUnits=deg  RotationMethod=AlignedAxes  RotationAngleUnits=deg  RotationStandardAxis=-Y  RotationAngle=180  RotationArbitraryAxis=[0 0 1]  FollAlignAxisA=+Y  BaseAlignAxisA=+Y  FollAlignAxisB=+X  BaseAlignAxisB=-X  RotationSequenceAxes=FollowerAxes  RotationSequence=XYX  RotationSequenceAngles=[0 0 0]  RotationSequenceAnglesUnits=deg  RotationMatrix=[1 0 0; 0 1 0; 0 0 1]
  Crank Arm : PMIOPort  Port=1  Side=Right
  Upper Arm : PMIOPort  Port=2  Side=Right
  connections:
  Bucket/RConn1 -- Attachment Frame/LConn1
  Crank Revolute Rotation/LConn1 -- Attachment Frame/RConn1
  Arm Revolute Rotation/LConn1 -- Attachment Frame/RConn2
  Upper Arm/RConn1 -- Arm Revolute Rotation/RConn1
  Crank Arm/RConn1 -- Crank Revolute Rotation/RConn1

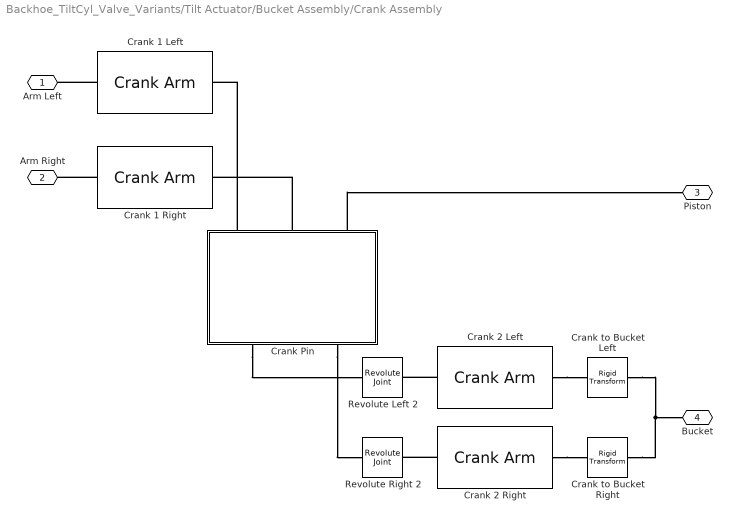
== system Backhoe_TiltCyl_Valve_Variants/Tilt Actuator/Bucket Assembly/Crank Assembly ==
  Crank 1 Left : Backhoe_Lib/Crank Arm  L=LC1  W=WC1  T=TC1  D=DH1  R=Rpin  Nc=25  color=color1  rho=rho1
  Crank 1 Right : Backhoe_Lib/Crank Arm  L=LC1  W=WC1  T=TC1  D=DH1  R=Rpin  Nc=25  color=color1  rho=rho1
  Crank 2 Left : Backhoe_Lib/Crank Arm  L=LC2  W=WC2  T=TC2  D=DH2  R=Rpin  Nc=25  color=color2  rho=rho2
  Crank 2 Right : Backhoe_Lib/Crank Arm  L=LC2  W=WC2  T=TC2  D=DH2  R=Rpin  Nc=25  color=color2  rho=rho2
  Crank Pin : Subsystem
      mask Display:
      | image(repmat(imread('Backhoe_Crankpin_IMAGE.png'),[1 1 3]));
      | port_label('lconn',1,'C1L');
      | port_label('lconn',2,'C2L');
      | port_label('lconn',3,'PA');
      | port_label('rconn',1,'C2L');
      | port_label('rconn',2,'C2R');
  Crank to Bucket Right : sm_lib/Frames and Transforms/Rigid Transform  TranslationMethod=StandardAxis  TranslationLengthUnit=m  TranslationStandardAxis=+Z  TranslationStandardOffset=(DC2 - TC2)/2  TranslationCartesianOffset=[0 0 0]  TranslationROffset=0  TranslationROffsetUnits=m  TranslationZOffset=0  TranslationZOffsetUnits=m  TranslationThetaOffset=0  TranslationThetaOffsetUnits=deg  RotationMethod=None  RotationAngleUnits=deg  RotationStandardAxis=+Z  RotationAngle=0  RotationArbitraryAxis=[0 0 1]  FollAlignAxisA=+X  BaseAlignAxisA=+Y  FollAlignAxisB=+Y  BaseAlignAxisB=+Z  RotationSequenceAxes=FollowerAxes  RotationSequence=XYX  RotationSequenceAngles=[0 0 0]  RotationSequenceAnglesUnits=deg  RotationMatrix=[1 0 0; 0 1 0; 0 0 1]
  Crank to Bucket Left : sm_lib/Frames and Transforms/Rigid Transform  TranslationMethod=StandardAxis  TranslationLengthUnit=m  TranslationStandardAxis=-Z  TranslationStandardOffset=(DC2 - TC2)/2  TranslationCartesianOffset=[0 0 0]  TranslationROffset=0  TranslationROffsetUnits=m  TranslationZOffset=0  TranslationZOffsetUnits=m  TranslationThetaOffset=0  TranslationThetaOffsetUnits=deg  RotationMethod=None  RotationAngleUnits=deg  RotationStandardAxis=+Z  RotationAngle=0  RotationArbitraryAxis=[0 0 1]  FollAlignAxisA=+X  BaseAlignAxisA=+Y  FollAlignAxisB=+Y  BaseAlignAxisB=+Z  RotationSequenceAxes=FollowerAxes  RotationSequence=XYX  RotationSequenceAngles=[0 0 0]  RotationSequenceAnglesUnits=deg  RotationMatrix=[1 0 0; 0 1 0; 0 0 1]
  Revolute Left 2 : sm_lib/Joints/Revolute Joint  SenseConstraintForce=off  SenseConstraintForceX=off  SenseConstraintForceY=off  SenseConstraintForceZ=off  SenseConstraintTorque=off  SenseConstraintTorqueX=off  SenseConstraintTorqueY=off  SenseConstraintTorqueZ=off  SenseTotalForce=off  SenseTotalForceX=off  SenseTotalForceY=off  SenseTotalForceZ=off  SenseTotalTorque=off  SenseTotalTorqueX=off  SenseTotalTorqueY=off  SenseTotalTorqueZ=off  CompositeWrenchDir=FollowerOnBase  CompositeWrenchFrame=BaseFrame  EquilibriumPosition=0  EquilibriumPositionUnits=deg  SpringStiffness=0  SpringStiffnessUnits=N*m/deg  DampingCoefficient=0  DampingCoefficientUnits=N*m/(deg/s)  TorqueActuationMode=NoTorque  MotionActuationMode=ComputedMotion  SensePosition=off  SenseVelocity=off  SenseAcceleration=off  SenseTorqueForce=off  PositionTargetSpecify=off  PositionTargetPriority=Low  PositionTargetValue=-45  PositionTargetValueUnits=deg  VelocityTargetSpecify=off  VelocityTargetPriority=High  VelocityTargetValue=0  VelocityTargetValueUnits=deg/s
  Revolute Right 2 : sm_lib/Joints/Revolute Joint  SenseConstraintForce=off  SenseConstraintForceX=off  SenseConstraintForceY=off  SenseConstraintForceZ=off  SenseConstraintTorque=off  SenseConstraintTorqueX=off  SenseConstraintTorqueY=off  SenseConstraintTorqueZ=off  SenseTotalForce=off  SenseTotalForceX=off  SenseTotalForceY=off  SenseTotalForceZ=off  SenseTotalTorque=off  SenseTotalTorqueX=off  SenseTotalTorqueY=off  SenseTotalTorqueZ=off  CompositeWrenchDir=FollowerOnBase  CompositeWrenchFrame=BaseFrame  EquilibriumPosition=0  EquilibriumPositionUnits=deg  SpringStiffness=0  SpringStiffnessUnits=N*m/deg  DampingCoefficient=0  DampingCoefficientUnits=N*m/(deg/s)  TorqueActuationMode=NoTorque  MotionActuationMode=ComputedMotion  SensePosition=off  SenseVelocity=off  SenseAcceleration=off  SenseTorqueForce=off  PositionTargetSpecify=off  PositionTargetPriority=High  PositionTargetValue=0  PositionTargetValueUnits=deg  VelocityTargetSpecify=off  VelocityTargetPriority=High  VelocityTargetValue=0  VelocityTargetValueUnits=deg/s
  Arm Left : PMIOPort  Port=1  Side=Left
  Arm Right : PMIOPort  Port=2  Side=Left
  Piston : PMIOPort  Port=3  Side=Right
  Bucket : PMIOPort  Port=4  Side=Right
  connections:
  Crank Pin/RConn1 -- Revolute Left 2/LConn1
  Crank Pin/RConn2 -- Revolute Right 2/LConn1
  Crank 2 Left/LConn1 -- Revolute Left 2/RConn1
  Crank to Bucket Right/RConn1 -- Crank to Bucket Left/RConn1 -- Bucket/RConn1
  Crank Pin/LConn3 -- Piston/RConn1
  Crank 1 Left/RConn1 -- Arm Left/RConn1
  Crank 1 Right/RConn1 -- Arm Right/RConn1
  Crank Pin/LConn1 -- Crank 1 Left/LConn1
  Crank Pin/LConn2 -- Crank 1 Right/LConn1
  Crank 2 Right/LConn1 -- Revolute Right 2/RConn1
  Crank 2 Right/RConn1 -- Crank to Bucket Right/LConn1
  Crank 2 Left/RConn1 -- Crank to Bucket Left/LConn1
